simulink model "cesna_a_37"  (Simulink 7.6)
settings: Solver=ode45  StartTime=0.0  StopTime=200  RelTol=1e-3
undefined symbols (not defined in the file or in its folder): A, alpha_trim, B, C, D, F_T_trim
libraries: simulink x3, Airframes x1
(part 2 of 2)

== system cesna_a_37/gamma_chi_controller/chi_controller/Hz_ipesh ==
  u : Inport
  Discrete State-Space : DiscreteStateSpace  A=A  B=B  C=C  D=D  X0=x0  SampleTime=Ts
  y : Outport
  wires:
  Discrete State-Space/1 -> y/1
  u/1 -> Discrete State-Space/1

== system cesna_a_37/omega_controller/alg_loop_filt/Hz_ipesh ==
  u : Inport
  Discrete State-Space : DiscreteStateSpace  A=A  B=B  C=C  D=D  X0=x0  SampleTime=Ts
  y : Outport
  wires:
  Discrete State-Space/1 -> y/1
  u/1 -> Discrete State-Space/1

== system cesna_a_37/omega_controller/alg_loop_filt/Hz_ipesh1 ==
  u : Inport
  Discrete State-Space : DiscreteStateSpace  A=A  B=B  C=C  D=D  X0=x0  SampleTime=Ts
  y : Outport
  wires:
  u/1 -> Discrete State-Space/1
  Discrete State-Space/1 -> y/1

== system cesna_a_37/omega_controller/alg_loop_filt/Hz_ipesh2 ==
  u : Inport
  Discrete State-Space : DiscreteStateSpace  A=A  B=B  C=C  D=D  X0=x0  SampleTime=Ts
  y : Outport
  wires:
  Discrete State-Space/1 -> y/1
  u/1 -> Discrete State-Space/1

== system cesna_a_37/omega_controller/omega_set_dot/Hz_ipesh ==
  u : Inport
  Discrete State-Space : DiscreteStateSpace  A=A  B=B  C=C  D=D  X0=x0  SampleTime=Ts
  y : Outport
  wires:
  Discrete State-Space/1 -> y/1
  u/1 -> Discrete State-Space/1

== system cesna_a_37/omega_controller/omega_set_dot/Hz_ipesh1 ==
  u : Inport
  Discrete State-Space : DiscreteStateSpace  A=A  B=B  C=C  D=D  X0=x0  SampleTime=Ts
  y : Outport
  wires:
  u/1 -> Discrete State-Space/1
  Discrete State-Space/1 -> y/1

== system cesna_a_37/omega_controller/omega_set_dot/Hz_ipesh2 ==
  u : Inport
  Discrete State-Space : DiscreteStateSpace  A=A  B=B  C=C  D=D  X0=x0  SampleTime=Ts
  y : Outport
  wires:
  Discrete State-Space/1 -> y/1
  u/1 -> Discrete State-Space/1

== system cesna_a_37/veocity_controller/anti_windup_control/Hz_ideal_plant ==
  u : Inport
  Discrete State-Space : DiscreteStateSpace  A=A  B=B  C=C  D=D  X0=x0  SampleTime=Ts
  y : Outport
  wires:
  Discrete State-Space/1 -> y/1
  u/1 -> Discrete State-Space/1

== matlab function alpha_beta_mu_controller/G_2_inverse ==
  settings: updateMethod=DISCRETE  sampleTime=Ts
  data: e input double; omega_d output double; alpha input double; rho input double; CLq parameter double; cbar parameter double; m parameter double; b parameter double; CYp parameter double; CYr parameter double; hat_x2 input double; G2_T_hat_x2 output double
function [omega_d,G2_T_hat_x2] = fcn(e, alpha, rho, CLq, cbar, m, b, CYp, CYr, hat_x2)
%#eml
c_22=1-(rho*CLq*cbar/(4*m));
c_31=(alpha+(b*rho*CYp/(4*m)));
c_33=-1+(b*rho*CYr/(4*m));
den=c_33 - (alpha*c_31);
G2_i=[c_33/den,0,-alpha/den;0,1/c_22,0;-c_31/den,0,1/den];
omega_d = G2_i*e;
G2=[1,0,alpha;0,c_22,0;c_31,0,c_33];
G2_T_hat_x2=G2' * hat_x2;

== matlab function gamma_chi_mu_sensor/Air Properties ==
  data: h input double; T output double; rho output double; g input double; ps output double; a output double
function [T,rho, ps, a] = fcn(h, g)
    %h altitude (meters)
    %g gravity at h (m/s^2)
    R = 8.31432; %J/(mol-Kelvin)
    M = 28.9644; %gm/mol
    To = 288.15; %standard temperature [Kelvin]
    Po = 101325; %standard pressure [Pa]
    L = 6.5; %Kelvin/km
    gamma = 1.4; %Gas constant for air
    T = To - 1.0e-3*L*h;            %Temperature at h
    ps = Po*(T/To)^((g*M)/(R*L));   %Pressure at h
    rho = ps/((1000*R/M)*T);        %Density at h
    a = sqrt(gamma*(R/(M*1e-3))*T); %speed of sound (m/s)

== matlab function omega_controller/Gamma_omega ==
  data: q_bar input double; Gamma_omega output double; omega input double; Clp parameter double; Clr parameter double; Cmq parameter double; Cnp parameter double; Cnr parameter double; S parameter double; b parameter double; cbar parameter double; V input double
function Gamma_omega = fcn(q_bar, omega, Clp, Clr, Cmq, Cnp, Cnr, S, b, cbar, V)
Gamma_omega=0*omega;
p=omega(1);
q=omega(2);
r=omega(3);
temp=q_bar*S/(2*V);
Gamma_omega(1)=temp*b*b*(Clp*p+Clr*r);
Gamma_omega(2)=temp*cbar*cbar*Cmq*q;
Gamma_omega(3)=temp*b*b*(Cnp*p+Cnr*r);

== matlab function omega_controller/w_cross_I_w ==
  data: u input double; y output double; I parameter double size=[3,3]
function y = fcn(u, I)
    p=u(1);
    q=u(2);
    r=u(3);
    w_cross = [0,-r,q;r,0,-p;-q,p,0];
    y = w_cross*I*u;
